simulink model "VDP_Sim_2014b"  (R2014b)
settings: Solver=FixedStepDiscrete  SolverMode=SingleTasking  StartTime=0.0  StopTime=max(t)  FixedStep=dt  RelTol=1e-3
values from neighbouring files (symbols this model uses):
  R = 1    [CDKF.m]    (also in estimator_demo.m = 0.2)
settings Model: CovMetricSettings=dwe  CovHtmlReporting=off  covSaveCumulativeToWorkspaceVar=off  CovSaveSingleToWorkspaceVar=off  CovExternalEMLEnable=on  CovSFcnEnable=on  Creator=BRUEN_T  LastModifiedBy=BRUEN_T
settings DataIOCC: LimitDataPoints=off  SaveFormat=StructureWithTime
settings DebuggingCC: SolverPrmCheckMsg=none  FrameProcessingCompatibilityMsg=error  SFUnexpectedBacktrackingDiag=error  SFNoUnconditionalDefaultTransitionDiag=error
settings HardwareCC: ProdBitPerPointer=64  ProdLargestAtomicFloat=Float  ProdIntDivRoundTo=Zero  ProdEndianess=LittleEndian  ProdHWDeviceType=Specified
settings ModelReferenceCC: PropagateSignalLabelsOutOfModel=on
settings GRTTargetCC: TargetLangStandard=C99 (ISO)  GeneratePreprocessorConditionals=Use local settings

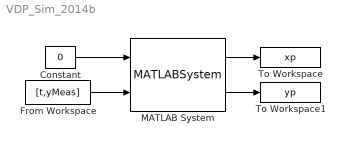
== system VDP_Sim_2014b ==
  Constant : Constant  Value=0
  From Workspace : FromWorkspace  VariableName=[t,yMeas]  SampleTime=0  OutputAfterFinalValue=Setting to zero
  MATLAB System : MATLABSystem  System=VDP_Estimator  mu=mu  x0=x0  Q=Q  R=R  P0=P0  h=sqrt( 3 )  dt=dt  SimulateUsing=Interpreted execution
      mask Type: VDP_Estimator
      mask Display:
      | disp('VDP_Estimator');
      | port_label('input',1,'u');
      | port_label('input',2,'y');
      | port_label('output',1,'xp');
      | port_label('output',2,'yp');
  To Workspace : ToWorkspace  VariableName=xp  SampleTime=-1
  To Workspace1 : ToWorkspace  VariableName=yp  SampleTime=-1
      settings: Save2DSignal=2-D array (concatenate along first dimension)
  wires:
  Constant/1 -> MATLAB System/1
  From Workspace/1 -> MATLAB System/2
  MATLAB System/1 -> To Workspace/1
  MATLAB System/2 -> To Workspace1/1
